simulink model "winter_simulink_IMM_control"  (R2022a)
settings: Solver=FixedStepAuto  StartTime=0  StopTime=stop_time  FixedStep=simulation.time_step_H
values from neighbouring files (symbols this model uses):
  B_eq = param{6}    [measurement_2states.m]    (also in measurement_2states_3mes.m; measurement_3measure.m)
  rho = param{2}    [measurement_3measure.m]
undefined symbols (not defined in the file or in its folder): blade, Gc, gearbox, generator, I_eq, IMM, lambda_vector, lookup_cP, omega_rated, P_est_initial, pitch_range, pitch_vector, rotor, T_R0, wind, wind_speed, x_est_initial
settings Model: Creator=Niccolò  LastModifiedBy=Niccolò
settings SolverCC: ZeroCrossAlgorithm=Adaptive
settings DebuggingCC: IgnoredZcDiagnostic=none

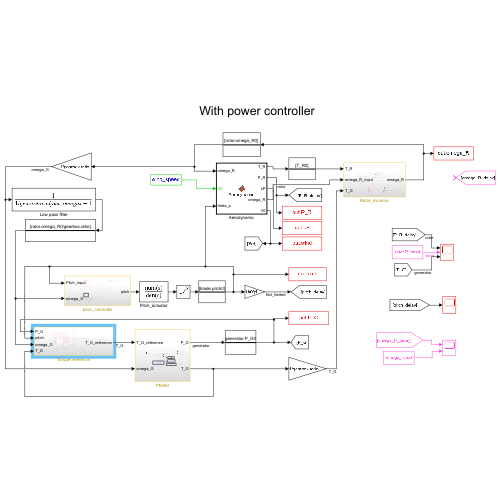
[thumbnail: Simulink's stored preview of the top-level diagram]
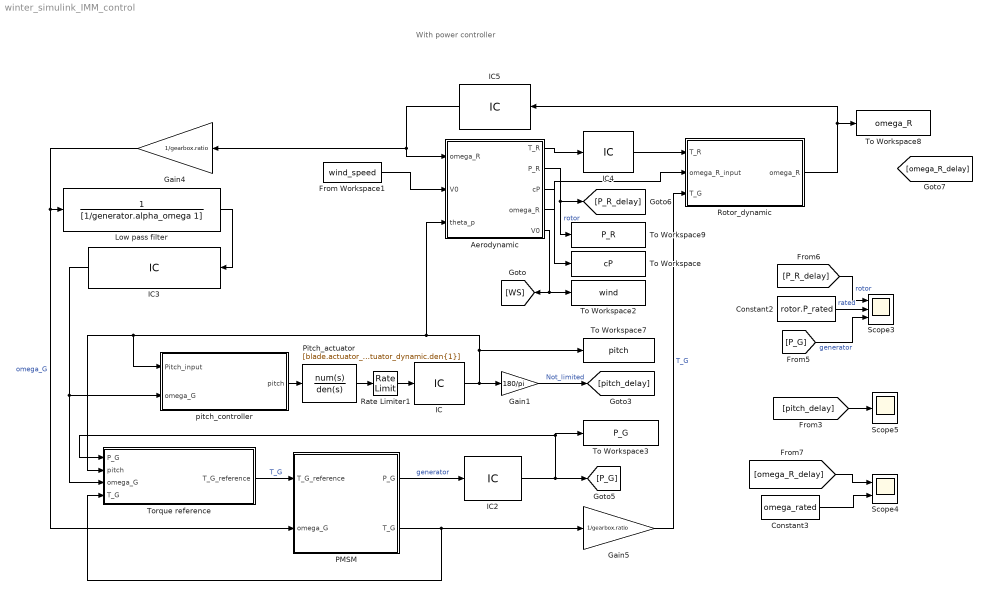
== system winter_simulink_IMM_control ==
  note: With power controller
  Aerodynamic : MATLAB Function  TreatAsAtomicUnit=on
  Constant2 : Constant  Value=rotor.P_rated
  Constant3 : Constant  Value=omega_rated
  From Workspace1 : FromWorkspace  VariableName=wind_speed  SampleTime=1/wind.sample_f
  Gain1 : Gain  Gain=180/pi
  Gain4 : Gain  Gain=1/gearbox.ratio
  Gain5 : Gain  Gain=1/gearbox.ratio
  IC : InitialCondition  Value=blade.pitch0
  IC2 : InitialCondition  Value=generator.P_G0
  IC3 : InitialCondition  Value=rotor.omega_R0/gearbox.ratio
  IC4 : InitialCondition  Value=T_R0
  IC5 : InitialCondition  Value=rotor.omega_R0
  Low pass filter : TransferFcn  Denominator=[1/generator.alpha_omega 1]
  PMSM : Subsystem
  Pitch_actuator : TransferFcn  Numerator=[blade.actuator_dynamic.num{1}]  Denominator=[blade.actuator_dynamic.den{1}]
  Rate Limiter1 : RateLimiter  RisingSlewLimit=blade.pitch_rate  FallingSlewLimit=-blade.pitch_rate  SampleTimeMode=inherited
  Rotor_dynamic : Subsystem
  Scope3 : Scope  NumInputPorts=3
  Scope4 : Scope  NumInputPorts=2
  Scope5 : Scope
  To Workspace : ToWorkspace  VariableName=cP  SaveFormat=Timeseries  SampleTime=-1
  To Workspace2 : ToWorkspace  VariableName=wind  SaveFormat=Timeseries  SampleTime=-1
  To Workspace3 : ToWorkspace  VariableName=P_G  SaveFormat=Timeseries  SampleTime=-1
  To Workspace7 : ToWorkspace  VariableName=pitch  SaveFormat=Timeseries  SampleTime=-1
  To Workspace8 : ToWorkspace  VariableName=omega_R  SaveFormat=Timeseries  SampleTime=-1
  To Workspace9 : ToWorkspace  VariableName=P_R  SaveFormat=Timeseries  SampleTime=-1
  Torque reference : Subsystem
  pitch_controller : Subsystem
  wires:
  From Workspace1/1 -> Aerodynamic/2("V0 ")
  Aerodynamic/2(P_R) -> To Workspace9/1, [P_R_delay]  "rotor"
  [pitch_delay] -> Scope5/1
  Gain4/1 -> PMSM/2(omega_G), Low pass filter/1  "omega_G"
  Rate Limiter1/1 -> IC/1
  [P_R_delay] -> Scope3/1  "rotor"
  Constant3/1 -> Scope4/2
  Constant2/1 -> Scope3/2  "rated"
  [omega_R_delay] -> Scope4/1
  Gain1/1 -> [pitch_delay]  "Not_limited"
  PMSM/2(T_G) -> Torque reference/4(T_G), Gain5/1
  Aerodynamic/1(T_R) -> IC4/1
  [P_G] -> Scope3/3  "generator"
  PMSM/1(P_G) -> IC2/1  "generator"
  pitch_controller/1(pitch) -> Pitch_actuator/1
  Pitch_actuator/1 -> Rate Limiter1/1
  Torque reference/1(T_G_reference) -> PMSM/1(T_G_reference)  "T_G"
  Gain5/1 -> Rotor_dynamic/3(T_G)  "T_G"
  IC/1 -> Gain1/1, To Workspace7/1, Aerodynamic/3(theta_p), Torque reference/2(pitch), pitch_controller/1(Pitch_input)
  IC3/1 -> pitch_controller/2(omega_G), Torque reference/3(omega_G)
  IC4/1 -> Rotor_dynamic/1(T_R)
  Rotor_dynamic/1(omega_R) -> IC5/1, To Workspace8/1
  IC5/1 -> Aerodynamic/1("omega_R "), Gain4/1
  Low pass filter/1 -> IC3/1
  IC2/1 -> To Workspace3/1, Torque reference/1(P_G), [P_G]
  Aerodynamic/4(omega_R) -> Rotor_dynamic/2(omega_R_input)
  Aerodynamic/3(cP) -> To Workspace/1
  Aerodynamic/5(V0) -> To Workspace2/1, [WS]

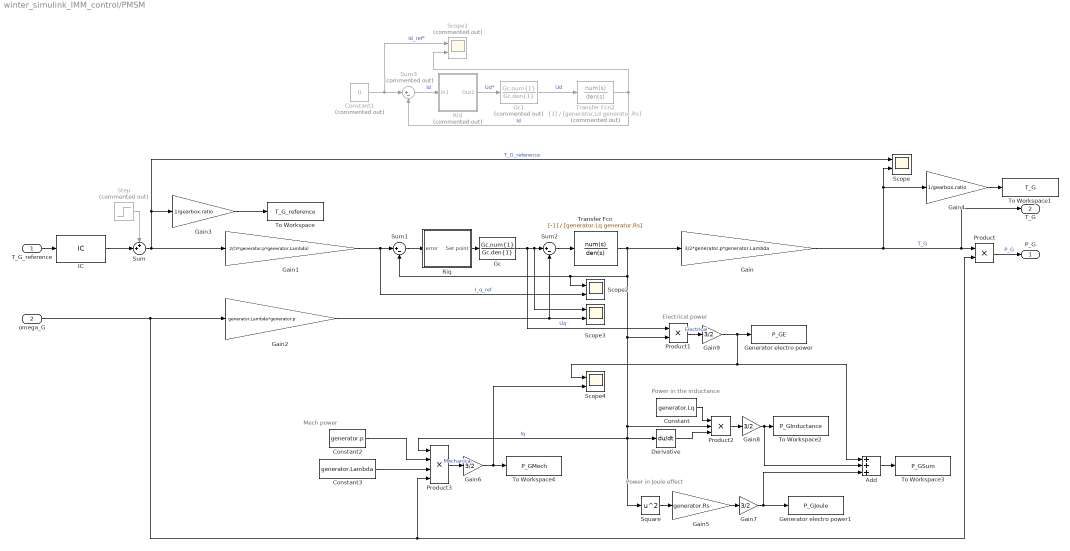
== system winter_simulink_IMM_control/PMSM ==
  note: Power in Joule effect
  note: Power in the inductance
  note: Electrical power
  note: Mech power
  T_G_reference : Inport
  omega_G : Inport  Port=2
  Add : Sum  Inputs=3
  Constant : Constant  Value=generator.Lq
  Constant1 : Constant  Commented=on  Value=0
  Constant2 : Constant  Value=generator.p
  Constant3 : Constant  Value=generator.Lambda
  Derivative : Derivative
  Gain : Gain  Gain=3/2*generator.p*generator.Lambda
  Gain1 : Gain  Gain=2/(3*generator.p*generator.Lambda)
  Gain2 : Gain  Gain=generator.Lambda*generator.p
  Gain3 : Gain  Gain=1/gearbox.ratio
  Gain4 : Gain  Gain=1/gearbox.ratio
  Gain5 : Gain  Gain=generator.Rs
  Gain{6..9} (4 alike) : Gain  Gain=3/2
  Gc : TransferFcn  Numerator=Gc.num{1}  Denominator=Gc.den{1}
  Gc1 : TransferFcn  Commented=on  Numerator=Gc.num{1}  Denominator=Gc.den{1}
  Generator electro power : ToWorkspace  VariableName=P_GE  SaveFormat=Timeseries  SampleTime=-1
  Generator electro power1 : ToWorkspace  VariableName=P_GJoule  SaveFormat=Timeseries  SampleTime=-1
  IC : InitialCondition  Value=generator.T_G0
  Product : Product
  Product1 : Product
  Product2 : Product  Inputs=3
  Product3 : Product  Inputs=4
  Rid : Subsystem  Commented=on
  Riq : Subsystem
  Scope{,2..4} (4 alike) : Scope  NumInputPorts=2
  Scope1 : Scope  Commented=on  NumInputPorts=2
  Square : Math  Operator=square
  Step : Step  Commented=on  Time=0.5  SampleTime=0
  Sum : Sum  Inputs=++|
  Sum1 : Sum  Inputs=|+-
  Sum2 : Sum  Inputs=|+-
  Sum3 : Sum  Commented=on  Inputs=|+-
  To Workspace : ToWorkspace  VariableName=T_G_reference  SaveFormat=Timeseries  SampleTime=-1
  To Workspace1 : ToWorkspace  VariableName=T_G  SaveFormat=Timeseries  SampleTime=-1
  To Workspace2 : ToWorkspace  VariableName=P_GInductance  SaveFormat=Timeseries  SampleTime=-1
  To Workspace3 : ToWorkspace  VariableName=P_GSum  SaveFormat=Timeseries  SampleTime=-1
  To Workspace4 : ToWorkspace  VariableName=P_GMech  SaveFormat=Timeseries  SampleTime=-1
  Transfer Fcn : TransferFcn  Numerator=[-1]  Denominator=[generator.Lq generator.Rs]
  Transfer Fcn2 : TransferFcn  Commented=on  Denominator=[generator.Ld generator.Rs]
  P_G : Outport
  T_G : Outport  Port=2
  wires:
  Gc/1 -> Product1/1, Scope3/1, Sum2/1  "Uq"
  Gain/1 -> T_G/1, Product/1, Gain4/1, Scope/2  "T_G"
  Riq/1(Set point) -> Gc/1
  Sum1/1 -> Riq/1(error)
  Transfer Fcn/1 -> Gain/1, Scope2/1, Sum1/2, Product1/2, Product3/1, Square/1, Derivative/1, Product2/2  "Iq"
  Product/1 -> P_G/1  "P_G"
  Gain1/1 -> Scope2/2, Sum1/1  "I_q_ref"
  Sum/1 -> Gain1/1, Scope/1, Gain3/1  "T_G_reference"
  T_G_reference/1 -> IC/1
  Step/1 -> Sum/1
  Sum2/1 -> Transfer Fcn/1
  Gain3/1 -> To Workspace/1
  IC/1 -> Sum/2
  Gain5/1 -> Gain7/1
  Square/1 -> Gain5/1
  Derivative/1 -> Product2/3
  Constant/1 -> Product2/1
  Product2/1 -> Gain8/1
  Gc1/1 -> Transfer Fcn2/1  "Ud"
  Rid/1(Out1) -> Gc1/1  "Ud*"
  Transfer Fcn2/1 -> Sum3/2, Scope1/2  "Id"
  Constant1/1 -> Scope1/1, Sum3/1  "Id_ref*"
  Sum3/1 -> Rid/1(In1)  "Id"
  Add/1 -> To Workspace3/1
  Constant2/1 -> Product3/2
  Constant3/1 -> Product3/3
  Product3/1 -> Gain6/1  "Mechanical"
  Product1/1 -> Gain9/1  "Electrical"
  Gain2/1 -> Scope3/2, Sum2/2
  omega_G/1 -> Product/2, Product3/4, Gain2/1
  Gain6/1 -> Scope4/2, To Workspace4/1
  Gain7/1 -> Generator electro power1/1, Add/3
  Gain8/1 -> To Workspace2/1, Add/2
  Gain9/1 -> Generator electro power/1, Add/1, Scope4/1
  Gain4/1 -> To Workspace1/1

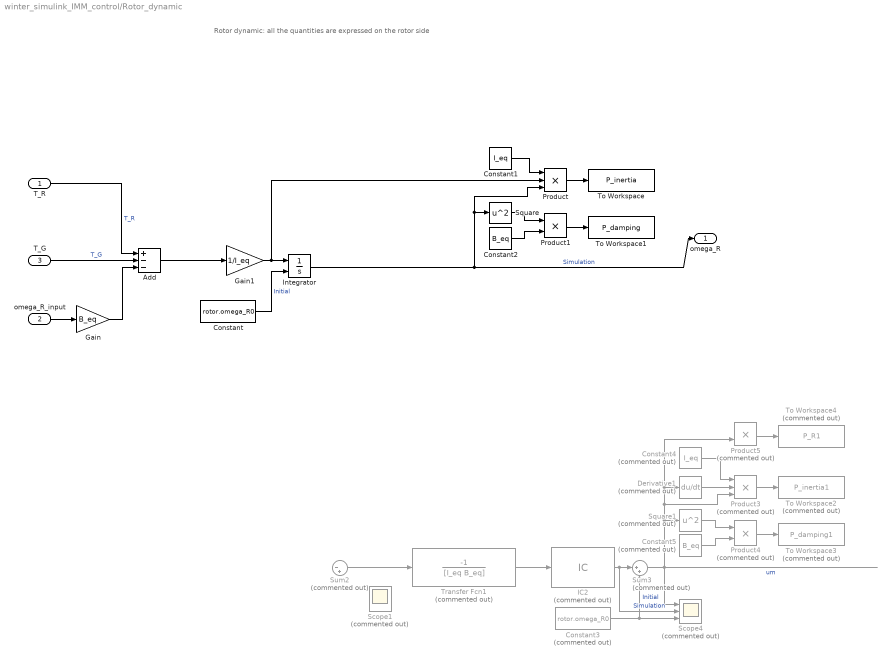
== system winter_simulink_IMM_control/Rotor_dynamic ==
  note: Rotor dynamic: all the quantities are expressed on the rotor side
  T_R : Inport
  omega_R_input : Inport  Port=2
  T_G : Inport  Port=3
  Add : Sum  Inputs=+--
  Constant : Constant  Value=rotor.omega_R0
  Constant1 : Constant  Value=I_eq
  Constant2 : Constant  Value=B_eq
  Constant3 : Constant  Commented=on  Value=rotor.omega_R0
  Constant4 : Constant  Commented=on  Value=I_eq
  Constant5 : Constant  Commented=on  Value=B_eq
  Derivative1 : Derivative  Commented=on
  Gain : Gain  Gain=B_eq
  Gain1 : Gain  Gain=1/I_eq
  IC2 : InitialCondition  Commented=on  Value=rotor.omega_R0
  Integrator : Integrator  InitialConditionSource=external
  Product : Product  Inputs=3
  Product1 : Product
  Product3 : Product  Commented=on  Inputs=3
  Product4 : Product  Commented=on
  Product5 : Product  Commented=on
  Scope1 : Scope  Commented=on  NumInputPorts=2
  Scope4 : Scope  Commented=on  NumInputPorts=3
  Square : Math  Operator=square
  Square1 : Math  Commented=on  Operator=square
  Sum2 : Sum  Commented=on  Inputs=|-+
  Sum3 : Sum  Commented=on  Inputs=|++
  To Workspace : ToWorkspace  VariableName=P_inertia  SaveFormat=Timeseries  SampleTime=-1
  To Workspace1 : ToWorkspace  VariableName=P_damping  SaveFormat=Timeseries  SampleTime=-1
  To Workspace2 : ToWorkspace  Commented=on  VariableName=P_inertia1  SaveFormat=Timeseries  SampleTime=-1
  To Workspace3 : ToWorkspace  Commented=on  VariableName=P_damping1  SaveFormat=Timeseries  SampleTime=-1
  To Workspace4 : ToWorkspace  Commented=on  VariableName=P_R1  SaveFormat=Timeseries  SampleTime=-1
  Transfer Fcn1 : TransferFcn  Commented=on  Numerator=[-1]  Denominator=[I_eq B_eq]
  omega_R : Outport
  wires:
  Integrator/1 -> Product/3, Square/1, omega_R/1  "Simulation"
  T_G/1 -> Add/2  "T_G"
  Constant/1 -> Integrator/2  "Initial"
  T_R/1 -> Add/1  "T_R"
  Add/1 -> Gain1/1
  Constant1/1 -> Product/1
  Product/1 -> To Workspace/1
  Constant2/1 -> Product1/2
  Product1/1 -> To Workspace1/1
  Square/1 -> Product1/1
  Square1/1 -> Product4/1
  Product5/1 -> To Workspace4/1
  Derivative1/1 -> Product3/2
  Product4/1 -> To Workspace3/1
  Constant4/1 -> Product3/1
  Constant5/1 -> Product4/2
  ? -> Scope1/2, Sum2/1, Product5/1  "T_R"
  ? -> Scope1/1, Sum2/2  "T_G"
  IC2/1 -> Scope4/2, Sum3/1  "Simulation"
  Sum2/1 -> Transfer Fcn1/1
  Product3/1 -> To Workspace2/1
  Transfer Fcn1/1 -> IC2/1
  Sum3/1 -> Product5/2, Derivative1/1, Product3/3, Square1/1, Scope4/1  "um"
  Constant3/1 -> Scope4/3, Sum3/2  "Initial"
  omega_R_input/1 -> Gain/1
  Gain/1 -> Add/3
  Gain1/1 -> Integrator/1, Product/2

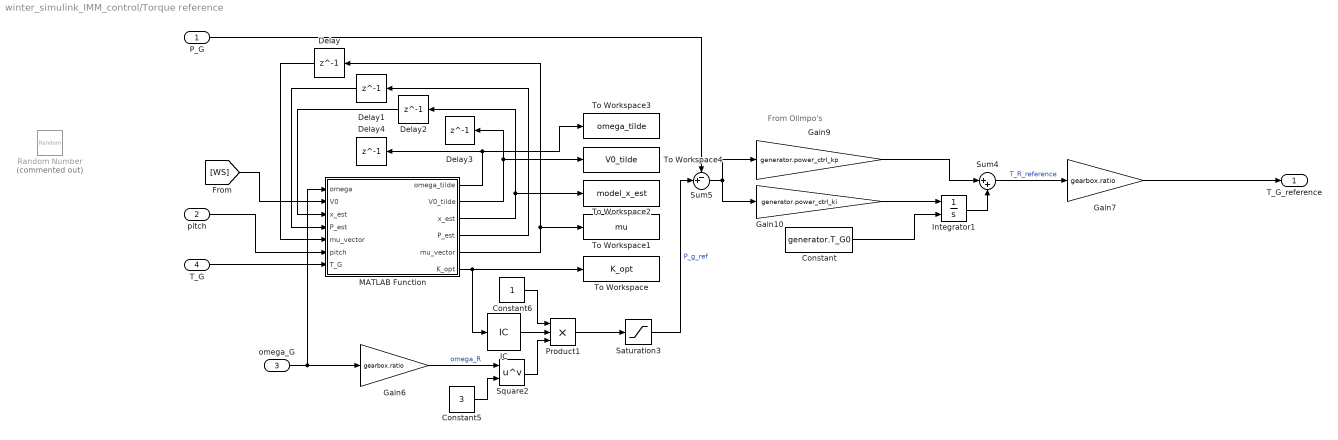
== system winter_simulink_IMM_control/Torque reference ==
  note: From Olimpo's
  P_G : Inport
  pitch : Inport  Port=2
  omega_G : Inport  Port=3
  T_G : Inport  Port=4
  Constant : Constant  Value=generator.T_G0
  Constant5 : Constant  Value=3
  Constant6 : Constant
  Delay : Delay  DelayLength=1  InitialCondition=ones(IMM.n_models, 1)/IMM.n_models
  Delay1 : Delay  DelayLength=1  InitialCondition=P_est_initial
  Delay2 : Delay  DelayLength=1  InitialCondition=x_est_initial
  Delay3 : Delay  DelayLength=1  InitialCondition=wind_speed(1, 2)
  Delay4 : Delay  DelayLength=1  InitialCondition=rotor.omega_R0
  Gain10 : Gain  Gain=generator.power_ctrl_ki
  Gain6 : Gain  Gain=gearbox.ratio
  Gain7 : Gain  Gain=gearbox.ratio
  Gain9 : Gain  Gain=generator.power_ctrl_kp
  IC : InitialCondition  Value=1e7
  Integrator1 : Integrator  InitialConditionSource=external
  MATLAB Function : MATLAB Function  TreatAsAtomicUnit=on
  Product1 : Product  Inputs=3
  Random Number : RandomNumber  Commented=on  Mean="[0  0]"  Variance=[1 1]  SampleTime=0.1  VectorParams1D=off
  Saturation3 : Saturate  UpperLimit=generator.P_rated  LowerLimit=0
  Square2 : Math  Operator=pow
  Sum4 : Sum  Inputs=|++
  Sum5 : Sum  Inputs=-+|
  To Workspace : ToWorkspace  VariableName=K_opt  SaveFormat=Timeseries  SampleTime=-1
  To Workspace1 : ToWorkspace  VariableName=mu  SaveFormat=Timeseries  SampleTime=-1
  To Workspace2 : ToWorkspace  VariableName=model_x_est  SaveFormat=Timeseries  SampleTime=-1
  To Workspace3 : ToWorkspace  VariableName=omega_tilde  SaveFormat=Timeseries  SampleTime=-1
  To Workspace4 : ToWorkspace  VariableName=V0_tilde  SaveFormat=Timeseries  SampleTime=-1
  T_G_reference : Outport
  wires:
  Square2/1 -> Product1/3
  Gain9/1 -> Sum4/1
  omega_G/1 -> MATLAB Function/1(omega), Gain6/1
  Gain10/1 -> Integrator1/1
  Constant/1 -> Integrator1/2
  Sum4/1 -> Gain7/1  "T_R_reference"
  Constant6/1 -> Product1/1
  Constant5/1 -> Square2/2
  Product1/1 -> Saturation3/1
  Gain6/1 -> Square2/1  "omega_R"
  Saturation3/1 -> Sum5/2  "P_g_ref"
  Integrator1/1 -> Sum4/2
  Sum5/1 -> Gain9/1, Gain10/1
  Gain7/1 -> T_G_reference/1
  P_G/1 -> Sum5/1
  MATLAB Function/6(K_opt) -> IC/1, To Workspace/1
  MATLAB Function/2(V0_tilde) -> To Workspace4/1, Delay3/1
  MATLAB Function/1(omega_tilde) -> To Workspace3/1, Delay4/1
  pitch/1 -> MATLAB Function/6(pitch)
  T_G/1 -> MATLAB Function/7(T_G)
  MATLAB Function/3(x_est) -> To Workspace2/1, Delay2/1
  MATLAB Function/4(P_est) -> Delay1/1
  MATLAB Function/5(mu_vector) -> To Workspace1/1, Delay/1
  Delay/1 -> MATLAB Function/5("mu_vector ")
  Delay1/1 -> MATLAB Function/4("P_est ")
  Delay2/1 -> MATLAB Function/3("x_est ")
  IC/1 -> Product1/2
  [WS] -> MATLAB Function/2(V0)

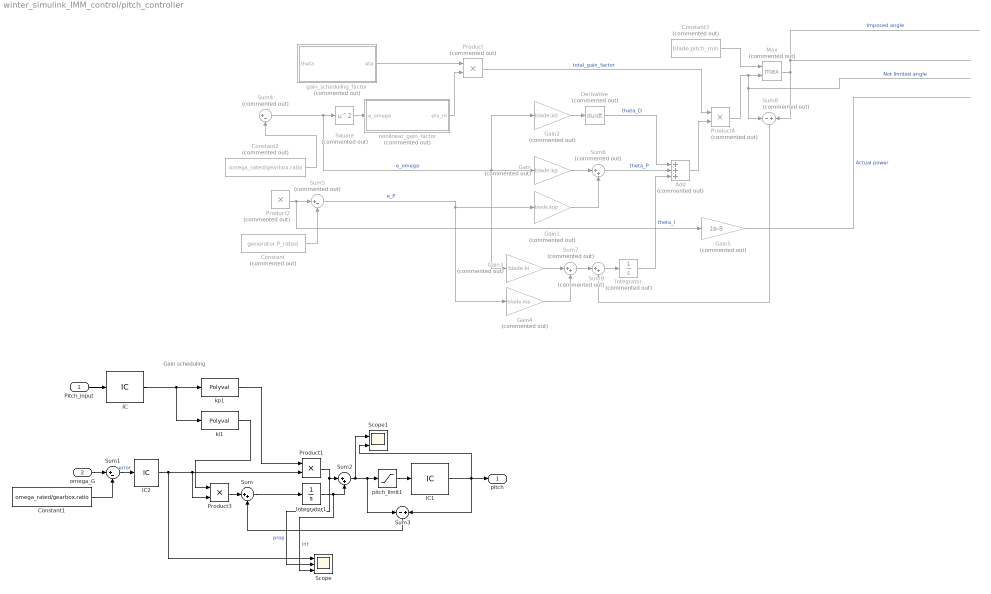
== system winter_simulink_IMM_control/pitch_controller ==
  note: Gain scheduling
  Pitch_input : Inport
  omega_G : Inport  Port=2
  Add : Sum  Commented=on  Inputs=+++
  Constant : Constant  Commented=on  Value=generator.P_rated
  Constant1 : Constant  Value=omega_rated/gearbox.ratio
  Constant2 : Constant  Commented=on  Value=omega_rated/gearbox.ratio
  Constant3 : Constant  Commented=on  Value=blade.pitch_min
  Derivative : Derivative  Commented=on
  Gain : Gain  Commented=on  Gain=blade.kp
  Gain1 : Gain  Commented=on  Gain=blade.kpp
  Gain2 : Gain  Commented=on  Gain=blade.kd
  Gain3 : Gain  Commented=on  Gain=blade.ki
  Gain4 : Gain  Commented=on  Gain=blade.kip
  Gain5 : Gain  Commented=on  Gain=1e-8
  IC : InitialCondition  Value=blade.pitch0
  IC1 : InitialCondition  Value=blade.pitch0
  IC2 : InitialCondition  Value=(rotor.omega_R0 - omega_rated)/gearbox.ratio
  Integrator : Integrator  Commented=on
  Integrator1 : Integrator
  Max : MinMax  Commented=on  Function=max  Inputs=2
  Product : Product  Commented=on
  Product1 : Product
  Product2 : Product  Commented=on
  Product3 : Product
  Product4 : Product  Commented=on
  Scope : Scope  NumInputPorts=3
  Scope1 : Scope  NumInputPorts=2
  Square : Math  Commented=on  Operator=square
  Sum : Sum  Inputs=|++
  Sum1 : Sum  Inputs=|+-
  Sum2 : Sum  Inputs=|++
  Sum3 : Sum  Inputs=-|+
  Sum4 : Sum  Commented=on  Inputs=|+-
  Sum5 : Sum  Commented=on  Inputs=|+-
  Sum6 : Sum  Commented=on  Inputs=|++
  Sum7 : Sum  Commented=on  Inputs=|++
  Sum8 : Sum  Commented=on  Inputs=-|+
  Sum9 : Sum  Commented=on  Inputs=|++
  gain_scheduling_factor : MATLAB Function  Commented=on  TreatAsAtomicUnit=on
  ki1 : Polyval  Coefs=blade.ki_schedule
  kp1 : Polyval  Coefs=blade.kp_schedule
  nonlinear_gain_factor : MATLAB Function  Commented=on  TreatAsAtomicUnit=on
  pitch_limit1 : Saturate  UpperLimit=pitch_range(2)  LowerLimit=0
  pitch : Outport
  wires:
  Sum/1 -> Integrator1/1
  Constant1/1 -> Sum1/2
  Product3/1 -> Sum/1
  omega_G/1 -> Sum1/1
  ki1/1 -> Product3/1
  kp1/1 -> Product1/1
  Sum1/1 -> IC2/1  "error"
  Product1/1 -> Scope/2, Sum2/1  "prop"
  Integrator1/1 -> Scope/3, Sum2/2  "int"
  ? -> ?  "Actual value"
  Sum8/1 -> Sum9/2
  Product4/1 -> Max/2, Sum8/1  "Not limited angle"
  Add/1 -> Product4/2
  Gain4/1 -> Sum7/2
  Product2/1 -> Gain5/1, Sum5/1
  Integrator/1 -> Add/3  "theta_I"
  ? -> Product2/2
  Derivative/1 -> Add/1  "theta_D"
  Product/1 -> Product4/1  "total_gain_factor"
  Sum6/1 -> Add/2  "theta_P"
  nonlinear_gain_factor/1(eta_nl) -> Product/2
  gain_scheduling_factor/1(eta) -> Product/1
  Gain/1 -> Sum6/1
  Max/1 -> Sum8/2  "Imposed angle"
  Sum5/1 -> Gain4/1, Gain1/1  "e_P"
  ? -> Sum4/1, Product2/1
  Constant2/1 -> Sum4/2
  Sum4/1 -> Gain3/1, Gain2/1, Gain/1, Square/1  "e_omega"
  Gain2/1 -> Derivative/1
  ? -> gain_scheduling_factor/1(theta)
  Gain5/1 -> ?  "Actual power"
  Constant/1 -> Sum5/2
  Constant3/1 -> Max/1
  Sum9/1 -> Integrator/1
  Gain1/1 -> Sum6/2
  Sum7/1 -> Sum9/1
  Square/1 -> nonlinear_gain_factor/1(e_omega)
  Gain3/1 -> Sum7/1
  Pitch_input/1 -> IC/1
  Sum2/1 -> pitch_limit1/1, Sum3/1, Scope1/1
  Sum3/1 -> Sum/2
  pitch_limit1/1 -> IC1/1
  IC/1 -> ki1/1, kp1/1
  IC1/1 -> Scope1/2, pitch/1, Sum3/2
  IC2/1 -> Scope/1, Product3/2, Product1/2

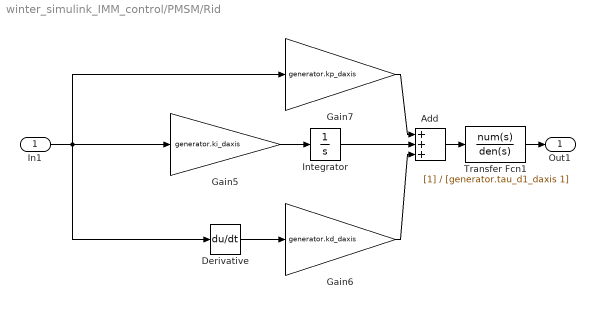
== system winter_simulink_IMM_control/PMSM/Rid ==
  In1 : Inport
  Add : Sum  Inputs=+++
  Derivative : Derivative
  Gain5 : Gain  Gain=generator.ki_daxis
  Gain6 : Gain  Gain=generator.kd_daxis
  Gain7 : Gain  Gain=generator.kp_daxis
  Integrator : Integrator
  Transfer Fcn1 : TransferFcn  Denominator=[generator.tau_d1_daxis 1]
  Out1 : Outport
  wires:
  Integrator/1 -> Add/2
  Add/1 -> Transfer Fcn1/1
  Gain7/1 -> Add/1
  Gain6/1 -> Add/3
  Derivative/1 -> Gain6/1
  In1/1 -> Derivative/1, Gain7/1, Gain5/1
  Transfer Fcn1/1 -> Out1/1
  Gain5/1 -> Integrator/1

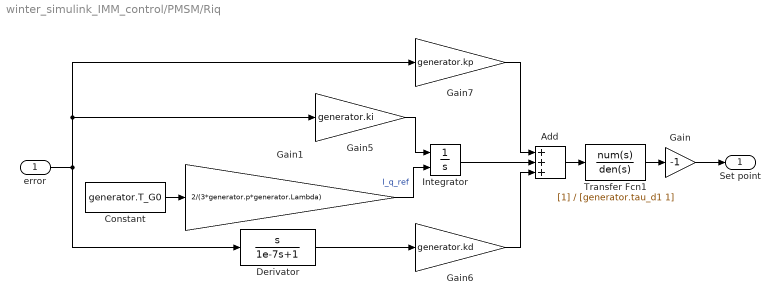
== system winter_simulink_IMM_control/PMSM/Riq ==
  error : Inport
  Add : Sum  Inputs=+++
  Constant : Constant  Value=generator.T_G0
  Derivator : TransferFcn  Numerator=[1 0]  Denominator=[1e-7 1]
  Gain : Gain  Gain=-1
  Gain1 : Gain  Gain=2/(3*generator.p*generator.Lambda)
  Gain5 : Gain  Gain=generator.ki
  Gain6 : Gain  Gain=generator.kd
  Gain7 : Gain  Gain=generator.kp
  Integrator : Integrator  InitialConditionSource=external
  Transfer Fcn1 : TransferFcn  Denominator=[generator.tau_d1 1]
  Set point : Outport
  wires:
  Integrator/1 -> Add/2
  Add/1 -> Transfer Fcn1/1
  Constant/1 -> Gain1/1
  Gain7/1 -> Add/1
  Gain6/1 -> Add/3
  Derivator/1 -> Gain6/1
  error/1 -> Gain5/1, Gain7/1, Derivator/1
  Transfer Fcn1/1 -> Gain/1
  Gain5/1 -> Integrator/1
  Gain1/1 -> Integrator/2  "I_q_ref"
  Gain/1 -> Set point/1

== matlab function winter_simulink_IMM_control/Aerodynamic ==
  data: omega_R input; V0 input; T_R output; P_R output; rho parameter; theta_p input; lambda_vector parameter; pitch_vector parameter; lookup_cP parameter; cP output; rotor parameter; omega_R output; V0 output
function [T_R, P_R, cP, omega_R, V0] = Aerodynamic(omega_R, V0, rho, theta_p, lambda_vector, pitch_vector, lookup_cP, rotor)

R = rotor.R;                  % rotor radius [m]

% retrive the cP from the look-up table
lambda = omega_R*R/V0;                                                
cP = interp2(lambda_vector, pitch_vector, lookup_cP, lambda, theta_p);

P_R = 0.5*rho*V0^3*pi*R^2*cP; % rotor power [W]
T_R = P_R/omega_R;            % rotor torque [Nm]

== matlab function winter_simulink_IMM_control/Torque reference/MATLAB Function ==
  settings: updateMethod=DISCRETE  sampleTime=simulation.time_step_H
  data: omega input; V0 input; x_est input size=[IMM.states_len, IMM.n_models]; P_est input size=[IMM.states_len, IMM.states_len, IMM.n_models]; mu_vector input size=[IMM.n_models, 1]; pitch input; T_G input; omega_tilde output size=1; V0_tilde output size=1; x_est output; P_est output; mu_vector output; K_opt output size=1; IMM parameter; I_eq parameter; rho parameter; rotor parameter; lambda_vector parameter; pitch_vector parameter; lookup_cP parameter
% This function wants to test the effectivness of the IMM for the estimation of the cp coefficient
function [omega_tilde, V0_tilde, x_est, P_est, mu_vector, K_opt] = gain_IMM(omega, V0, x_est, P_est, mu_vector, pitch, T_G, IMM, I_eq, rho, rotor, lambda_vector , pitch_vector, lookup_cP)
% x_est -> (states_len, n_models) items containing the state estimation
% P_est -> (states_len, states_len, n_models) containing the covariance

n_models = IMM.n_models; % number of models to test
states_len = IMM.states_len; % length of the states
Pi = IMM.Pi; 
R = IMM.R;
Q = IMM.Q;
cp_vector = IMM.cp_vector;
mu = zeros(n_models);
% Vector of parameters
param = cell(6,1);
param{1} = I_eq;
param{2} = rho;
param{3} = rotor.R;
param{4} = 0;
param{5} = R;
param{6} = Q;
x_real = [omega; V0];
omega_tilde = 0;

% Assamble the model cell
model = cell(n_models, 1);
for j=1:n_models
  model{j} = struct('cp', IMM.cp_vector(j), 'x_est', x_est(1:states_len, j), 'P_est', P_est(1:states_len,1:states_len,j), 'z_hat', 0, 'P_prior', P_est(1:states_len,1:states_len,j), 'Lambda', 0, 'mu', mu_vector(j), 'mu_new', 0, 'x_tilde', zeros(states_len, 1), 'P_tilde', zeros(states_len));
end

% Simulate the measurement
z = measurement(x_real, param{5}) + my_mvnrnd([0], R, 1)'; % rotational speed measurement [rad/s]

% Filtering
model = filtering(model, z, T_G, param);

% Output estimation
model = output_estimation(model, param);

% Mode probability updating
model = probability_updating(model, z, param);

% State combination
x_est_g = zeros(states_len, 1); % global state
[x_est_g(1:states_len, 1), ~] = state_combination(model);
omega_tilde = x_est_g(1); % estimation of the rotational speed
V0_tilde = x_est_g(2); % estimation of the wind speed
% Filter interaction
[model, model_prob] = filter_interaction(model, Pi);
[~, idx] = max(model_prob); % model with the highest probability

% Compute the gain
% K_opt = 0.5*IMM.cp_vector(idx)*pi*param{2}*param{3}^2*x_est_g(2)^3/x_est_g(1)^3;
K_opt = 0.5*IMM.cp_vector(idx)*pi*param{2}*param{3}^2/7.4^3;

% Assemble the model cell
for j=1:n_models
  x_est(1:states_len, j) = model{j}.x_est(1:states_len);
  P_est(1:states_len,1:states_len,j) = model{j}.P_est(1:states_len, 1:states_len);
  mu_vector(j) = model{j}.mu_new(1);
end

end

%   _____ _  _______ 
%  | ____| |/ /  ___|
%  |  _| | ' /| |_   
%  | |___| . \|  _|  
%  |_____|_|\_\_|    
                   
function [model] = EKF(model, z, T_G, param, matrices)
  % y -> measurement of the rotational speed [rad/s]
  
  x_est = model.x_est;
  P_est = model.P_est;

  F = matrices.F;
  H = matrices.H;
  Q = matrices.Q;
  R = matrices.R;
  G = matrices.G;

  % Prediction
  x_est = dynamic(x_est(1:2), T_G, param);
  P_est = F*P_est*F' + G*Q*G';
  P_prior = P_est;
  states_len = size(x_est, 1); % number of states

  % Update
  [~, z_hat] = measurement(x_est, param{5}); % estimation of the measurement using the sensor's model
  Innovation = z - z_hat;
  S_Inno = H*P_est*H' + R;
  W = P_est*H'*inv(S_Inno); % kalman gain
  x_est = x_est + W*Innovation; % update state estimate
  P_est = (eye(states_len) - W*H)*P_est; % update covariance matrix


  model.x_est(1:states_len) = x_est(1:states_len);
  model.P_est(1:states_len, 1:states_len) = P_est(1:states_len, 1:states_len);
  model.z_hat = z_hat;
  model.P_prior = P_prior;
end

%   ____                              _      
%  |  _ \ _   _ _ __   __ _ _ __ ___ (_) ___ 
%  | | | | | | | '_ \ / _` | '_ ` _ \| |/ __|
%  | |_| | |_| | | | | (_| | | | | | | | (__ 
%  |____/ \__, |_| |_|\__,_|_| |_| |_|_|\___|
%         |___/                              

function x_new = dynamic(x_est, T_G, param)

  I_eq = param{1}; % Inertia
  rho = param{2}; % Density
  R = param{3}; % Radius
  cp = param{4}; % Power coefficient
  x_new = zeros(2,1);

  x_new(1) = x_est(1) + 1/I_eq*(1/2*rho*pi*R^2*cp*x_est(2)^3*x_est(1)^(-1) - T_G);
  x_new(2) = x_est(2);
end

%   __  __                                                    _   
%  |  \/  | ___  __ _ ___ _   _ _ __ ___ _ __ ___   ___ _ __ | |_ 
%  | |\/| |/ _ \/ _` / __| | | | '__/ _ \ '_ ` _ \ / _ \ '_ \| __|
%  | |  | |  __/ (_| \__ \ |_| | | |  __/ | | | | |  __/ | | | |_ 
%  |_|  |_|\___|\__,_|___/\__,_|_|  \___|_| |_| |_|\___|_| |_|\__|
                                     
function [z, z_hat] = measurement(x, R)
  % z_hat -> fake measuerement to be used in the KF

  z_hat = x(1); % rotational speed [rad/s]
  z = x(1); %+ mvnrnd([0], R)'; % rotational speed [rad/s]
end

%    ____                            _                         _     
%   / ___|___  _ __ ___  _ __  _   _| |_ ___   _ __ ___   __ _| |_   
%  | |   / _ \| '_ ` _ \| '_ \| | | | __/ _ \ | '_ ` _ \ / _` | __|  
%  | |__| (_) | | | | | | |_) | |_| | ||  __/ | | | | | | (_| | |_ _ 
%   \____\___/|_| |_| |_| .__/ \__,_|\__\___| |_| |_| |_|\__,_|\__(_)
%                       |_|                                          

function matrices = compute_matrices(x_est, param)

  I_eq = param{1}; % Inertia
  rho = param{2}; % Density
  R = param{3}; % Radius
  cp = param{4}; % Power coefficient

  F = [1-1/I_eq*(1/2*rho*pi*R^2*cp*x_est(2)^3*x_est(1)^(-2)) 1/I_eq*(3/2*rho*pi*R^2*cp*x_est(2)^2*x_est(1)^(-1));
       0 1];
  H = [1 0];
  G = [1 1];
%   matrices = cell(4, 1);
  matrices = struct('F', F, 'H', H, 'G', G);
end

%   _____ _ _ _            _             
%  |  ___(_) | |_ ___ _ __(_)_ __   __ _ 
%  | |_  | | | __/ _ \ '__| | '_ \ / _` |
%  |  _| | | | ||  __/ |  | | | | | (_| |
%  |_|   |_|_|\__\___|_|  |_|_| |_|\__, |
%                                  |___/ 

function model = filtering(model, z, T_G, param)
  n_models = size(model, 1);
  for j=1:n_models
    param{4} = model{j}.cp;
    % compute the linearized matrices
    matrices = compute_matrices(model{j}.x_est(1:2), param);
    matrices.R = param{5};
    matrices.Q = param{6};

    [model{j}] = EKF(model{j}, z, T_G, param, matrices);
  end
end

%   ____            _                       _       _   _             
%  |  _ \ _ __ ___ | |__    _   _ _ __   __| | __ _| |_(_)_ __   __ _ 
%  | |_) | '__/ _ \| '_ \  | | | | '_ \ / _` |/ _` | __| | '_ \ / _` |
%  |  __/| | | (_) | |_) | | |_| | |_) | (_| | (_| | |_| | | | | (_| |
%  |_|   |_|  \___/|_.__/   \__,_| .__/ \__,_|\__,_|\__|_|_| |_|\__, |
%                                |_|                            |___/ 

function model = probability_updating(model, z, param)
  n_models = size(model, 1);
  for j=1:n_models
    % compute the linearized matrices
    matrices = compute_matrices(model{j}.x_est, param);
    matrices.R = param{5};
    matrices.Q = param{6}; 
    H = matrices.H;
    R = matrices.R;
    G = matrices.G;
    z_hat = model{j}.z_hat;
    P_prior = model{j}.P_prior;

    S = H*P_prior*H' + G*R*G';
    zeta = z - z_hat;
    model{j}.Lambda = 1/sqrt(2*pi*det(S))*exp(-1/2*zeta'*inv(S)*zeta);
  end
  % Compute the denominator
  den = 0;
  for j=1:n_models
    den = den + model{j}.mu*model{j}.Lambda;
  end
  % Update model probability
  for j=1:n_models
    model{j}.mu = model{j}.mu*model{j}.Lambda/den;
  end
end

%   ____  _        _                             _      
%  / ___|| |_ __ _| |_ ___    ___ ___  _ __ ___ | |__   
%  \___ \| __/ _` | __/ _ \  / __/ _ \| '_ ` _ \| '_ \  
%   ___) | || (_| | ||  __/ | (_| (_) | | | | | | |_) | 
%  |____/ \__\__,_|\__\___|  \___\___/|_| |_| |_|_.__(_)
                                                      
function [x_est, P_est] = state_combination(model)
  n_models = size(model, 1);
  states_len = size(model{1}.x_est, 1);
  x_est = zeros(states_len,1);
  P_est = zeros(states_len,states_len);
  for j=1:n_models
    x_est(1:states_len) = x_est(1:states_len) + model{j}.mu*model{j}.x_est(1:states_len);
  end
  
  for j=1:n_models
    P_est = P_est + model{j}.mu*(model{j}.P_est + (x_est - model{j}.x_est)*(x_est - model{j}.x_est)');
  end

end

%   _____ _ _ _              _       _                      _   _             
%  |  ___(_) | |_ ___ _ __  (_)_ __ | |_ ___ _ __ __ _  ___| |_(_) ___  _ __  
%  | |_  | | | __/ _ \ '__| | | '_ \| __/ _ \ '__/ _` |/ __| __| |/ _ \| '_ \ 
%  |  _| | | | ||  __/ |    | | | | | ||  __/ | | (_| | (__| |_| | (_) | | | |
%  |_|   |_|_|\__\___|_|    |_|_| |_|\__\___|_|  \__,_|\___|\__|_|\___/|_| |_|
                                                                            
function [model, model_prob] = filter_interaction(model, Pi)
  n_models = size(model, 1);
  states_len = size(model{1}.x_est, 1);
  mu = zeros(n_models, n_models);

  for j=1:n_models
    model{j}.mu_new = 0;
    for i=1:n_models
        model{j}.mu_new = model{j}.mu_new + Pi(i, j)*model{i}.mu; 
    end
  end

  for j=1:n_models
    for i=1:n_models
        mu(i, j) = Pi(i, j)*model{i}.mu/model{j}.mu_new;
    end
  end

  for j=1:n_models
    model{j}.x_tilde(1:states_len, 1) = zeros(states_len, 1);
    model{j}.P_tilde = zeros(states_len, states_len);
    for i=1:n_models
      model{j}.x_tilde = model{j}.x_tilde + mu(i, j)*model{i}.x_est;
    end
    for i=1:n_models
        model{j}.P_tilde = model{j}.P_tilde + mu(i, j)*(model{i}.P_est + (model{j}.x_tilde - model{i}.x_est)*(model{j}.x_tilde - model{i}.x_est)');
    end
    model{j}.x_est = model{j}.x_tilde;
    model{j}.P_est = model{j}.P_tilde;
  end

  % Store the value of the probability
  model_prob = zeros(n_models, 1);
  for j=1:n_models
    model_prob(j) = model{j}.mu_new;
  end
end

%    ___        _               _               _     
%   / _ \ _   _| |_ _ __  _   _| |_    ___  ___| |_   
%  | | | | | | | __| '_ \| | | | __|  / _ \/ __| __|  
%  | |_| | |_| | |_| |_) | |_| | |_  |  __/\__ \ |_ _ 
%   \___/ \__,_|\__| .__/ \__,_|\__|  \___||___/\__(_)
%                  |_|                                

function model = output_estimation(model, param)
  n_models = size(model, 1);
  R = param{3}; % Radius
  lambda = 0;
  for j=1:n_models
    x_est_1 = model{j}.x_est(1);
    x_est_2 = model{j}.x_est(2);
    lambda = R*x_est_1/x_est_2; 
  end
end

%                                       _ 
%   _ __ _____   ___ __  _ __ _ __   __| |
%  | '_ ` _ \ \ / / '_ \| '__| '_ \ / _` |
%  | | | | | \ V /| | | | |  | | | | (_| |
%  |_| |_| |_|\_/ |_| |_|_|  |_| |_|\__,_|
                                        
function y = my_mvnrnd(mu, cov, n)
    % Cholesky decomposition
    L = chol(cov, 'lower');

    % Generate standard normal random numbers
    z = randn(n, length(mu));

    % Transform to multivariate normal
    y = L*z' + mu;

    y = y';
end

== matlab function winter_simulink_IMM_control/pitch_controller/gain_scheduling_factor ==
  data: eta output; theta input; blade parameter
function eta = gain_scheduling_factor(theta, blade)

K1 = blade.K1;
K2 = blade.K2;

theta = theta*180/pi; % [deg]

eta = 1/(1+ theta/K1 + theta^2/K2);

== matlab function winter_simulink_IMM_control/pitch_controller/nonlinear_gain_factor ==
  data: e_omega input; eta_nl output; blade parameter; generator parameter
function eta_nl = nonlinear_gain_factor(e_omega, blade, generator)

omega_rated = generator.omega_rated;
omega2 = omega_rated*blade.omega2omega0ratio;

eta_nl = 1 + e_omega^2/(omega2 - omega_rated)^2;
